simulink model "task3"  (R2024a)
settings: Solver=FixedStepAuto  StartTime=0.0  StopTime=10.0  FixedStep=15  RelTol=1e-15
settings Model: Creator=kit  LastModifiedBy=kit

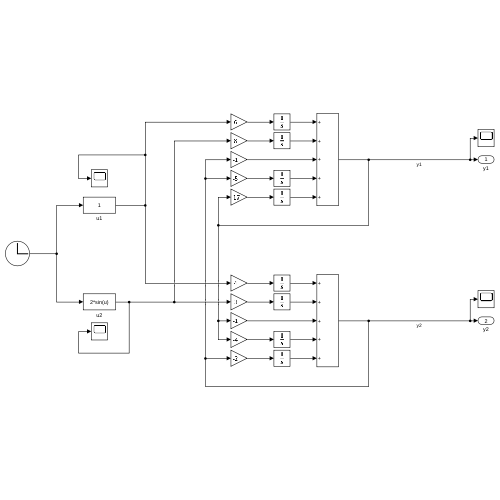
[thumbnail: Simulink's stored preview of the top-level diagram]
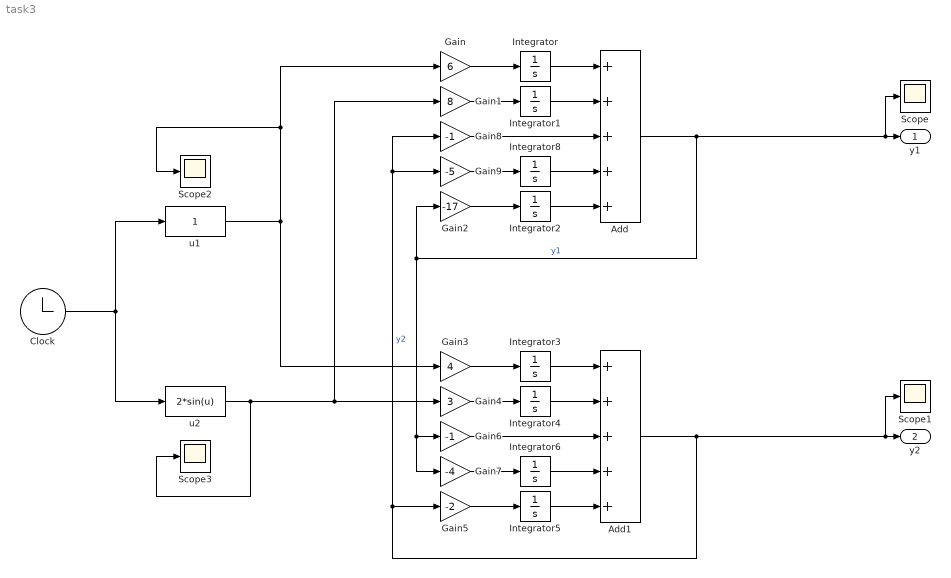
== system task3 ==
  Add : Sum  Inputs=+++++
  Add1 : Sum  Inputs=+++++
  Clock : Clock
  Gain : Gain  Gain=6
  Gain1 : Gain  Gain=8
  Gain2 : Gain  Gain=-17
  Gain3 : Gain  Gain=4
  Gain4 : Gain  Gain=3
  Gain5 : Gain  Gain=-2
  Gain6 : Gain  Gain=-1
  Gain7 : Gain  Gain=-4
  Gain8 : Gain  Gain=-1
  Gain9 : Gain  Gain=-5
  Integrator{,1..6,8} (8 alike) : Integrator
  Scope{,1..3} (4 alike) : Scope
  u1 : Fcn  Expr=1
  u2 : Fcn  Expr=2*sin(u)
  y1 : Outport
  y2 : Outport  Port=2
  wires:
  Clock/1 -> u2/1, u1/1
  u1/1 -> Gain3/1, Scope2/1, Gain/1
  Gain/1 -> Integrator/1
  Integrator/1 -> Add/1
  Integrator1/1 -> Add/2
  Gain1/1 -> Integrator1/1
  u2/1 -> Gain4/1, Gain1/1, Scope3/1
  Add/1 -> Scope/1, y1/1, Gain7/1, Gain6/1, Gain2/1  "y1"
  Gain2/1 -> Integrator2/1
  Integrator2/1 -> Add/5
  Gain4/1 -> Integrator4/1
  Add1/1 -> Scope1/1, y2/1, Gain5/1, Gain8/1, Gain9/1  "y2"
  Gain5/1 -> Integrator5/1
  Integrator3/1 -> Add1/1
  Integrator5/1 -> Add1/5
  Integrator4/1 -> Add1/2
  Gain3/1 -> Integrator3/1
  Gain6/1 -> Add1/3
  Gain7/1 -> Integrator6/1
  Integrator6/1 -> Add1/4
  Gain8/1 -> Add/3
  Gain9/1 -> Integrator8/1
  Integrator8/1 -> Add/4
